simulink subsystem "JoystickInitializer"  (R2023a)
settings: Solver=VariableStepAuto  StartTime=0.0  StopTime=10.0  RelTol=1e-3
settings Model: Creator=yzk0058  LastModifiedBy=gcs-comp2

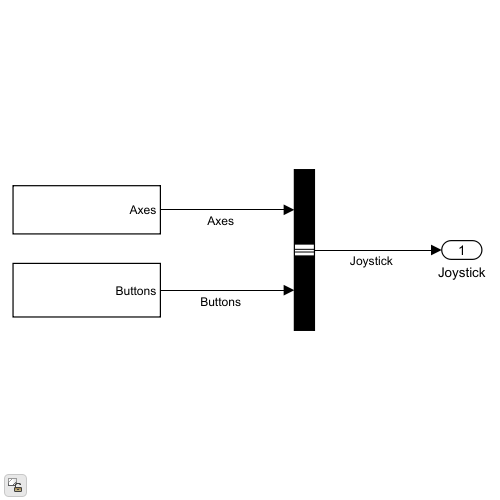
[thumbnail: Simulink's stored preview of the top-level diagram]
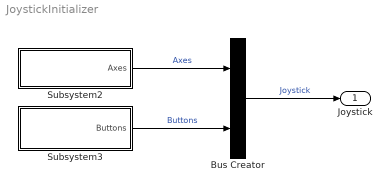
== system JoystickInitializer ==
  Bus Creator : BusCreator  Inputs=2
  Subsystem2 : Subsystem
  Subsystem3 : Subsystem
  Joystick : Outport
  wires:
  Subsystem3/1(Buttons) -> Bus Creator/2  "Buttons"
  Subsystem2/1(Axes) -> Bus Creator/1  "Axes"
  Bus Creator/1 -> Joystick/1  "Joystick"

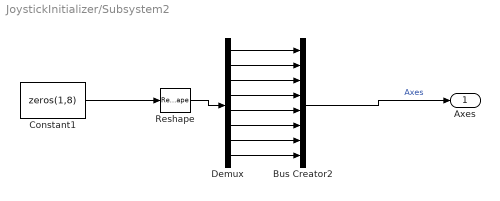
== system JoystickInitializer/Subsystem2 ==
  Bus Creator2 : BusCreator  Inputs=8
  Constant1 : Constant  Value=zeros(1,8)
  Demux : Demux  Outputs=8
  Reshape : Reshape
  Axes : Outport
  wires:
  Demux/8 -> Bus Creator2/8
  Demux/7 -> Bus Creator2/7
  Demux/6 -> Bus Creator2/6
  Demux/5 -> Bus Creator2/5
  Constant1/1 -> Reshape/1
  Demux/2 -> Bus Creator2/2
  Reshape/1 -> Demux/1
  Bus Creator2/1 -> Axes/1  "Axes"
  Demux/1 -> Bus Creator2/1
  Demux/4 -> Bus Creator2/4
  Demux/3 -> Bus Creator2/3

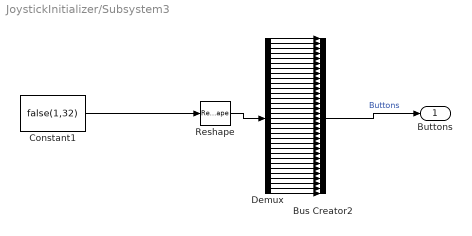
== system JoystickInitializer/Subsystem3 ==
  Bus Creator2 : BusCreator  Inputs=32
  Constant1 : Constant  Value=false(1,32)  OutDataTypeStr=boolean
  Demux : Demux  Outputs=32
  Reshape : Reshape
  Buttons : Outport
  wires:
  Demux/32 -> Bus Creator2/32
  Demux/31 -> Bus Creator2/31
  Demux/30 -> Bus Creator2/30
  Demux/29 -> Bus Creator2/29
  Demux/28 -> Bus Creator2/28
  Demux/27 -> Bus Creator2/27
  Demux/26 -> Bus Creator2/26
  Constant1/1 -> Reshape/1
  Demux/25 -> Bus Creator2/25
  Demux/24 -> Bus Creator2/24
  Demux/23 -> Bus Creator2/23
  Demux/22 -> Bus Creator2/22
  Demux/21 -> Bus Creator2/21
  Demux/20 -> Bus Creator2/20
  Demux/19 -> Bus Creator2/19
  Demux/18 -> Bus Creator2/18
  Demux/17 -> Bus Creator2/17
  Demux/16 -> Bus Creator2/16
  Demux/15 -> Bus Creator2/15
  Demux/14 -> Bus Creator2/14
  Demux/13 -> Bus Creator2/13
  Demux/12 -> Bus Creator2/12
  Demux/11 -> Bus Creator2/11
  Demux/10 -> Bus Creator2/10
  Demux/9 -> Bus Creator2/9
  Demux/8 -> Bus Creator2/8
  Demux/7 -> Bus Creator2/7
  Demux/6 -> Bus Creator2/6
  Demux/5 -> Bus Creator2/5
  Demux/3 -> Bus Creator2/3
  Demux/4 -> Bus Creator2/4
  Demux/1 -> Bus Creator2/1
  Bus Creator2/1 -> Buttons/1  "Buttons"
  Reshape/1 -> Demux/1
  Demux/2 -> Bus Creator2/2
